simulink model "Simple_4Quad_payload_03"  (R2018b)
settings: Solver=VariableStepAuto  StartTime=0.0  StopTime=60  RelTol=1e-3
InitFcn:
  | Simple_4Quad_payload_03_const
values from neighbouring files (symbols this model uses):
  B = 1e0*eye(n)    [Simple_2Quad_payload_03_const.m]    (also in constant_CAMFC2_Quad_New_02_Payload_01.m = eye(n); test01.m = [eye(3) eye(3) eye(3) eye(3))
  BBT_inv = ((B'*B)^(-1))*B'    [Simple_2Quad_payload_03_const.m]    (also in Simple_4Quad_payload_04_const.m = ((BR'*BR)^(-1))*BR'; Simple_4Quad_payload_05_const.m = ((BR'*BR)^(-1))*BR'; Simple_4Quad_payload_06_const.m = ((BR'*BR)^(-1))*BR'; Simple_4Quad_payload_07_const.m = ((BR'*BR)^(-1))*BR')
  d1 = 0.25    [Colab_4Quad_model_01_const.m]    (also in Colab_4Quad_model_02_const.m = 0.5; Simple_4Quad_payload_01_const.m = 1; Simple_4Quad_payload_02_const.m = 1; Simple_4Quad_payload_03_const.m = 1)
  d2 = 0.25    [Colab_4Quad_model_01_const.m]    (also in Colab_4Quad_model_02_const.m = 0.5; Simple_4Quad_payload_01_const.m = 1; Simple_4Quad_payload_02_const.m = 1; Simple_4Quad_payload_03_const.m = 1)
  Des_rel_dist = 2    [Simple_4Quad_payload_01_const.m]    (also in Simple_4Quad_payload_02_const.m = 4; Simple_4Quad_payload_03_const.m = 4; Simple_4Quad_payload_04_const.m; Simple_4Quad_payload_05_const.m)
  gamma_0 = 1e-0*diag([1e-3;1e-0])    [Simple_2Quad_payload_03_const.m]    (also in Simple_4Quad_payload_04_const.m = 1e-0*diag([1e-6*ones(3,1);1e-0*ones(3,1)]); Simple_4Quad_payload_05_const.m = 1e-1*diag([1e-6*ones(3,1);1e-0*ones(3,1)]); Simple_4Quad_payload_06_const.m = 1e-0*diag([1e-6*ones(3,1);1e-0*ones(3,1)]); Simple_4Quad_payload_07_const.m = 1e-0*diag([1e-6*ones(3,1);1e-0*ones(3,1)]))
  gamma_1 = 1e+2*diag([1e-3;1e-0])    [Simple_2Quad_payload_03_const.m]    (also in Simple_4Quad_payload_04_const.m = 1e+2*diag([1e-6*ones(3,1);1e-0*ones(3,1)]); Simple_4Quad_payload_05_const.m = 1e+2*diag([1e-6*ones(3,1);1e-0*ones(3,1)]); Simple_4Quad_payload_06_const.m = 1e+3*diag([1e-6*ones(3,1);1e-0*ones(3,1)]); Simple_4Quad_payload_07_const.m = 1e+3*diag([1e-6*ones(3,1);1e-0*ones(3,1)]))
  ge = 9.81    [Simple_4Quad_payload_03_const.m]    (also in constant_CAMFC2_Quad_New_02_Payload_01.m)
  Ix = 0.166667    [Colab_4Quad_model_01_const.m]    (also in Colab_4Quad_model_02_const.m = 0.02; Simple_4Quad_payload_01_const.m = 1; Simple_4Quad_payload_02_const.m = 1; Simple_4Quad_payload_03_const.m = 1)
  Iy = 0.166667    [Colab_4Quad_model_01_const.m]    (also in Colab_4Quad_model_02_const.m = 0.02; Simple_4Quad_payload_01_const.m = 1; Simple_4Quad_payload_02_const.m = 1; Simple_4Quad_payload_03_const.m = 1)
  Iz = 0.166667    [Colab_4Quad_model_01_const.m]    (also in Colab_4Quad_model_02_const.m = 0.02; Simple_4Quad_payload_01_const.m = 1; Simple_4Quad_payload_02_const.m = 1; Simple_4Quad_payload_03_const.m = 1)
  Jq = diag([0.0291 0.0291 0.0552])    [Colab_4Quad_model_01_const.m]    (also in Colab_4Quad_model_02_const.m = diag([0.03 0.03 0.06]); Simple_4Quad_payload_03_const.m = 1.2416e-3 * diag([1 1 2]); Simple_4Quad_payload_04_const.m = 1 * diag([1 1 2]); Simple_4Quad_payload_05_const.m = 1 * diag([1 1 2]))
  k1 = 1    [Simple_2Quad_payload_03_const.m]    (also in Simple_4Quad_payload_04_const.m; Simple_4Quad_payload_05_const.m; Simple_4Quad_payload_06_const.m; Simple_4Quad_payload_07_const.m)
  k2 = 0.1    [Simple_2Quad_payload_03_const.m]    (also in Simple_4Quad_payload_04_const.m; Simple_4Quad_payload_05_const.m; Simple_4Quad_payload_06_const.m; Simple_4Quad_payload_07_const.m)
  Ka = 0.01    [Simple_4Quad_payload_03_const.m]    (also in constant_CAMFC2_Quad_New_02_Payload_01.m)
  Kd = 0.01    [Simple_4Quad_payload_03_const.m]    (also in constant_CAMFC2_Quad_New_02_Payload_01.m)
  Kf = 1.0e-5    (= 1e-05)    [Simple_4Quad_payload_03_const.m]    (also in constant_CAMFC2_Quad_New_02_Payload_01.m)
  ki1_N = 0    [Simple_4Quad_payload_02_const.m]    (also in Simple_4Quad_payload_03_const.m; Simple_4Quad_payload_04_const.m; Simple_4Quad_payload_05_const.m; Simple_4Quad_payload_06_const.m)
  ki1_S = 0    [Simple_4Quad_payload_02_const.m]    (also in Simple_4Quad_payload_03_const.m; Simple_4Quad_payload_04_const.m)
  ki2_N = 0    [Simple_4Quad_payload_02_const.m]    (also in Simple_4Quad_payload_03_const.m; Simple_4Quad_payload_04_const.m; Simple_4Quad_payload_05_const.m; Simple_4Quad_payload_06_const.m = 10)
  ki2_S = 0    [Simple_4Quad_payload_02_const.m]    (also in Simple_4Quad_payload_03_const.m; Simple_4Quad_payload_04_const.m)
  kp1_N = 10    [Simple_4Quad_payload_02_const.m]    (also in Simple_4Quad_payload_03_const.m; Simple_4Quad_payload_04_const.m; Simple_4Quad_payload_05_const.m = 1; Simple_4Quad_payload_06_const.m = 1)
  kp1_S = 10    [Simple_4Quad_payload_02_const.m]    (also in Simple_4Quad_payload_03_const.m; Simple_4Quad_payload_04_const.m)
  kp2_N = 100    [Simple_4Quad_payload_02_const.m]    (also in Simple_4Quad_payload_03_const.m; Simple_4Quad_payload_04_const.m; Simple_4Quad_payload_05_const.m = 1; Simple_4Quad_payload_06_const.m = 1)
  kp2_S = 100    [Simple_4Quad_payload_02_const.m]    (also in Simple_4Quad_payload_03_const.m; Simple_4Quad_payload_04_const.m)
  Kt = 0.0435 * Kf    (= 4.35e-07)    [Simple_4Quad_payload_03_const.m]    (also in constant_CAMFC2_Quad_New_02_Payload_01.m = 1e-07)
  l = 3.1819    [Colab_4Quad_model_01_const.m]    (also in Colab_4Quad_model_02_const.m = 3; Simple_2Quad_payload_04_const.m = 1; Simple_4Quad_payload_01_const.m = 1; Simple_4Quad_payload_02_const.m = 2)
  Lq = 0.45    [Simple_4Quad_payload_03_const.m]    (also in constant_CAMFC2_Quad_New_02_Payload_01.m = 0.2)
  m = 1.5    [Colab_4Quad_model_01_const.m]    (also in Colab_4Quad_model_02_const.m; Simple_2Quad_payload_04_const.m = 1; Simple_4Quad_payload_01_const.m = 1; Simple_4Quad_payload_02_const.m = 1)
  M = 1.0    (= 1)    [Colab_4Quad_model_01_const.m]    (also in Colab_4Quad_model_02_const.m; Simple_2Quad_payload_01_const.m; Simple_2Quad_payload_02_const.m; Simple_2Quad_payload_03_const.m)
  Md = 1*[1;1;1]    [Simple_2Quad_payload_04_const.m]    (also in Simple_4Quad_payload_01_const.m = 1*[1;1;1;1;1;1]; Simple_4Quad_payload_02_const.m = 1*[1;1;1;1;1;1]; Simple_4Quad_payload_03_const.m = 1*[1;1;1;1;1;1]; Simple_4Quad_payload_04_const.m = 1*[1;1;1;1;1;1])
  Mq = 2.95    [Simple_4Quad_payload_03_const.m]
  n = 2    [Simple_2Quad_payload_03_const.m]    (also in Simple_4Quad_payload_03_const.m = 6; Simple_4Quad_payload_04_const.m = 6; Simple_4Quad_payload_05_const.m = 6; Simple_4Quad_payload_06_const.m = 6)
  QR = 1e-0*eye(n)    [Simple_4Quad_payload_04_const.m]    (also in Simple_4Quad_payload_05_const.m = 1e-1*eye(n); Simple_4Quad_payload_06_const.m; Simple_4Quad_payload_07_const.m; Simple_4Quad_payload_08_const.m)
  R = 1e+0*eye(n)    [Simple_2Quad_payload_03_const.m]    (also in Simple_4Quad_payload_04_const.m = 1e+0*eye(m); Simple_4Quad_payload_05_const.m = 1e+0*eye(m); Simple_4Quad_payload_06_const.m; Simple_4Quad_payload_07_const.m)
  rho_0 = 1e-0    (= 1)    [Simple_2Quad_payload_03_const.m]    (also in Simple_4Quad_payload_04_const.m; Simple_4Quad_payload_05_const.m = 0.1; Simple_4Quad_payload_06_const.m; Simple_4Quad_payload_07_const.m)
  rho_1 = 1e-0    (= 1)    [Simple_2Quad_payload_03_const.m]    (also in Simple_4Quad_payload_04_const.m; Simple_4Quad_payload_05_const.m; Simple_4Quad_payload_06_const.m; Simple_4Quad_payload_07_const.m)
undefined symbols (not defined in the file or in its folder): mq
libraries: simulink x16
(part 3 of 3)

== matlab function Simple_4Quad_payload_03/Agent2/Quadrotor Plant #2/MATLAB Function ==
  data: XT2 input; XR2 input; Omega2_des input; t input; D_XT2 output; Kf parameter; Kt parameter; Kd parameter; Ka parameter; Mq parameter; Jq parameter; Lq parameter; ge parameter; D_XR2 output
function [D_XT2,D_XR2] = fcn(XT2,XR2,Omega2_des,t,Kf,Kt,Kd,Ka,Mq,Jq,Lq,ge)

phi_2 = XR2(1);
theta_2 = XR2(2);
psi_2 = XR2(3);

Rq_2 = [cos(psi_2)*cos(theta_2) -sin(psi_2)*cos(phi_2)+cos(psi_2)*sin(theta_2)*sin(phi_2) sin(psi_2)*sin(phi_2)+cos(psi_2)*sin(theta_2)*cos(phi_2);
    sin(psi_2)*cos(theta_2) cos(psi_2)*cos(phi_2)+sin(psi_2)*sin(theta_2)*sin(phi_2) -cos(psi_2)*sin(phi_2)+sin(psi_2)*sin(theta_2)*cos(phi_2);
    -sin(theta_2) cos(theta_2)*sin(phi_2) cos(theta_2)*cos(phi_2)]; 

R_omega_2 = [1 0 -sin(theta_2);
    0 cos(phi_2) cos(theta_2)*sin(phi_2);
    0 -sin(phi_2) cos(theta_2)*cos(phi_2)];

EXT_PRD_2 = External_Product3(XR2(4:6),(Jq*XR2(4:6)));

F1_2 = Kf * Omega2_des(1)^2;
F2_2 = Kf * Omega2_des(2)^2;
F3_2 = Kf * Omega2_des(3)^2;
F4_2 = Kf * Omega2_des(4)^2;
  
FT_2 = F1_2 + F2_2 + F3_2 + F4_2;
 
T1_2 = Kt * Omega2_des(1)^2;
T2_2 = Kt * Omega2_des(2)^2;
T3_2 = Kt * Omega2_des(3)^2;
T4_2 = Kt * Omega2_des(4)^2;
 
TT1_2 = Lq*(F3_2 - F1_2);
TT2_2 = Lq*(F4_2 - F2_2);
TT3_2 = (T1_2 - T2_2 + T3_2 - T4_2);

FTT_2 = Rq_2 * [0;0;FT_2];
FTx_2 = FTT_2(1);
FTy_2 = FTT_2(2);
FTz_2 = FTT_2(3);

DP_2 = XT2(4:6);
DPHI_2 = (R_omega_2)^(-1) * XR2(4:6); 
Dv_2 = (1/Mq)*([FTx_2;FTy_2;FTz_2] - Kd*XT2(4:6) - Mq*[0;0;ge]) + Rq_2*(0.0*sin(1*t))*[0;0;1]; 
Dw_2 = (Jq^(-1))*([TT1_2;TT2_2;TT3_2] - Ka*XR2(4:6) - EXT_PRD_2) + (0*sin(1*t)*[1;1;1]);

D_XT2 = [DP_2;Dv_2];
D_XR2 = [DPHI_2;Dw_2];

end

== matlab function Simple_4Quad_payload_03/Agent3/Attitude Controller #3/Rotational #3/CARE ==
  data: P input; a_hat input; B parameter; R parameter; DP output; QR parameter
function DP = fcn(P,a_hat,B,R,QR)

DP = a_hat*P + P*a_hat' - P*B*R*B'*P + 2*QR;

end

== matlab function Simple_4Quad_payload_03/Agent3/Attitude Controller #3/Rotational #3/Differentiator/Sliding differentiator ==
  data: u output; u1 input; e input; n parameter; k1 parameter
function u = fcn(u1,e,n,k1)

b=k1;

ABS = zeros(n,1);
for i=1:n
    if e(i)>0
        ABS(i) = e(i);
    else
        ABS(i) = -e(i);
    end
end
SGN = e ./ (ABS + 0.01);

u = u1 - b*(ABS.^0.5).*SGN;

end

== matlab function Simple_4Quad_payload_03/Agent3/Attitude Controller #3/Rotational #3/Differentiator/Sliding differentiator1 ==
  data: Du1 output; e input; n parameter; k2 parameter
function Du1 = fcn(e,n,k2)

a=k2;

ABS = zeros(n,1);
for i=1:n
    if e(i)>0
        ABS(i) = e(i);
    else
        ABS(i) = -e(i);
    end
end
SGN = e ./ (ABS + 0.01);

Du1 = - a*SGN;

end

== matlab function Simple_4Quad_payload_03/Agent3/Attitude Controller #3/Rotational #3/g-Estimator ==
  data: sigma input; g_hat input; P input; rho_1 parameter; gamma_1 parameter; Dg_hat output
function Dg_hat = fcn(sigma,g_hat,P,rho_1,gamma_1)

Dg_hat = - gamma_1 * P * sigma - rho_1 * gamma_1 * g_hat;

end

== matlab function Simple_4Quad_payload_03/Agent3/Attitude Controller #3/Rotational #3/g-Estimator1 ==
  data: sigma input; x input; P input; rho_0 parameter; gamma_0 parameter; Da_hat output; a_hat input
function Da_hat = fcn(sigma,x,P,rho_0,gamma_0,a_hat)

DVa_hat = - gamma_0 * P * diag(sigma) * (x - sigma) - rho_0 * gamma_0 * diag(a_hat);

Da_hat = diag(DVa_hat);

end

== matlab function Simple_4Quad_payload_03/Agent3/Attitude Controller #3/Rotational #3/main ==
  data: sigma input; zeta input; u output; Dy_d input; R parameter; P input; a_hat input; B parameter; g_hat input; x input; QR parameter; BBT_inv parameter; n parameter
function u = fcn(sigma,zeta,Dy_d,R,P,a_hat,B,g_hat,x,QR,BBT_inv,n)

u1 = (1/2) * R * B' * P * sigma;
u2 = BBT_inv * (Dy_d - a_hat*x + (eye(n) + 2*(((P)^(-1)*QR)) + a_hat)*sigma - g_hat - zeta) - (3/4) * R * B' * P * sigma;

u = u1 + u2;

end

== matlab function Simple_4Quad_payload_03/Agent3/Attitude Controller #3/Rotational #3/variable change ==
  data: X input; Xd input; x_mod output; u input; xd_mod output; e_mod output
function [x_mod,xd_mod,e_mod] = fcn(X,Xd,u)

x_mod = [X(4:6);X(10:12)];

xd_mod = [Xd;u(1:3)];

e_mod = xd_mod - x_mod;


end

== matlab function Simple_4Quad_payload_03/Agent3/Link angle computation #3 ==
  data: XT3 input; Alpha_act_3 output; Po input; Beta_act_3 output; PHIo input; L_meas_3 output
function [Alpha_act_3,Beta_act_3,L_meas_3] = fcn(XT3,Po,PHIo)

phi = PHIo(1);
theta = PHIo(2);
psi = PHIo(3);

Ro = [cos(psi)*cos(theta) cos(psi)*sin(theta)*sin(phi)-sin(psi)*cos(phi) cos(psi)*sin(theta)*cos(phi)+sin(psi)*sin(phi);
    sin(psi)*cos(theta) sin(psi)*sin(theta)*sin(phi)+cos(psi)*cos(phi) sin(psi)*sin(theta)*cos(phi)-cos(psi)*sin(phi);
    -sin(theta) cos(theta)*sin(phi) cos(theta)*cos(phi)];

P_diff_3 = Ro' * ( XT3(1:3) - Po );

L_meas_3 = sqrt( (P_diff_3(1)^2) + (P_diff_3(2)^2) + (P_diff_3(3)^2) );
Alpha_act_3 = asin( P_diff_3(3)/L_meas_3 );
Beta_act_3 = atan2( P_diff_3(2),P_diff_3(1) );
if Beta_act_3 < (-3*pi/4)
    Beta_act_3 = 2*pi + Beta_act_3;
end



end

== matlab function Simple_4Quad_payload_03/Agent3/Link dynamic Model #3 ==
  data: N3 input; S3 input; f3 input; alpha_3 input; beta_3 input; D_alpha_3 input; D_beta_3 input; mq parameter; ge parameter; DD_PHIo input; DD_Po input; D_PHIo input; l parameter; d2 parameter; PHIo input; U3_des output; Po input; P3_des output
function [U3_des,P3_des] = fcn(N3,S3,f3,alpha_3,beta_3,D_alpha_3,D_beta_3,mq,ge,DD_PHIo,DD_Po,D_PHIo, l, d2,PHIo,Po)

phi = PHIo(1);
theta = PHIo(2);
psi = PHIo(3);

Dist3_local = [0;+d2;0];
D3_angles = [0;D_alpha_3;D_beta_3];

Ro = [cos(psi)*cos(theta) cos(psi)*sin(theta)*sin(phi)-sin(psi)*cos(phi) cos(psi)*sin(theta)*cos(phi)+sin(psi)*sin(phi);
    sin(psi)*cos(theta) sin(psi)*sin(theta)*sin(phi)+cos(psi)*cos(phi) sin(psi)*sin(theta)*cos(phi)-cos(psi)*sin(phi);
    -sin(theta) cos(theta)*sin(phi) cos(theta)*cos(phi)];

R3 = [cos(alpha_3)*cos(beta_3) -sin(beta_3) -sin(alpha_3)*cos(beta_3);
    cos(alpha_3)*sin(beta_3) cos(beta_3) -sin(alpha_3)*sin(beta_3);
    sin(alpha_3) 0 cos(alpha_3)];

C1_3 = External_Product3(D_PHIo,Dist3_local);
C2_3 = External_Product3(D_PHIo,C1_3);
C3_3 = External_Product3(DD_PHIo,Dist3_local);
C4_3 = External_Product3(D3_angles,Dist3_local);
C5_3 = External_Product3(D3_angles,C4_3);

a3_part = (  R3' * ( Ro'*DD_Po + C2_3 + C3_3 ) ) + C5_3;
G3_local = R3' * Ro' * [0;0;-ge];

T3 = mq*a3_part(1) + f3 - mq*G3_local(1);
U3_des = Ro * R3 * [T3;S3;N3];

%DD_alpha3 = (1/mq/l) * (N3 - mq*a3_part(2) + mq*G3_local(2));
%DD_beta3 = (1/mq/l) * (S3 - mq*a3_part(3) + mq*G3_local(3));
P3_des = Po + Ro*Dist3_local + Ro*R3*[l;0;0];

end

== matlab function Simple_4Quad_payload_03/Agent3/Quadrotor Plant #3/MATLAB Function ==
  data: XT3 input; XR3 input; Omega3_des input; t input; D_XT3 output; Kf parameter; Kt parameter; Kd parameter; Ka parameter; Mq parameter; Jq parameter; Lq parameter; ge parameter; D_XR3 output
function [D_XT3,D_XR3] = fcn(XT3,XR3,Omega3_des,t,Kf,Kt,Kd,Ka,Mq,Jq,Lq,ge)

phi_3 = XR3(1);
theta_3 = XR3(2);
psi_3 = XR3(3);

Rq_3 = [cos(psi_3)*cos(theta_3) -sin(psi_3)*cos(phi_3)+cos(psi_3)*sin(theta_3)*sin(phi_3) sin(psi_3)*sin(phi_3)+cos(psi_3)*sin(theta_3)*cos(phi_3);
    sin(psi_3)*cos(theta_3) cos(psi_3)*cos(phi_3)+sin(psi_3)*sin(theta_3)*sin(phi_3) -cos(psi_3)*sin(phi_3)+sin(psi_3)*sin(theta_3)*cos(phi_3);
    -sin(theta_3) cos(theta_3)*sin(phi_3) cos(theta_3)*cos(phi_3)]; 

R_omega_3 = [1 0 -sin(theta_3);
    0 cos(phi_3) cos(theta_3)*sin(phi_3);
    0 -sin(phi_3) cos(theta_3)*cos(phi_3)];

EXT_PRD_3 = External_Product3(XR3(4:6),(Jq*XR3(4:6)));

F1_3 = Kf * Omega3_des(1)^2;
F2_3 = Kf * Omega3_des(2)^2;
F3_3 = Kf * Omega3_des(3)^2;
F4_3 = Kf * Omega3_des(4)^2;
  
FT_3 = F1_3 + F2_3 + F3_3 + F4_3;
 
T1_3 = Kt * Omega3_des(1)^2;
T2_3 = Kt * Omega3_des(2)^2;
T3_3 = Kt * Omega3_des(3)^2;
T4_3 = Kt * Omega3_des(4)^2;
 
TT1_3 = Lq*(F3_3 - F1_3);
TT2_3 = Lq*(F4_3 - F2_3);
TT3_3 = (T1_3 - T2_3 + T3_3 - T4_3);

FTT_3 = Rq_3 * [0;0;FT_3];
FTx_3 = FTT_3(1);
FTy_3 = FTT_3(2);
FTz_3 = FTT_3(3);

DP_3 = XT3(4:6);
DPHI_3 = (R_omega_3)^(-1) * XR3(4:6); 
Dv_3 = (1/Mq)*([FTx_3;FTy_3;FTz_3] - Kd*XT3(4:6) - Mq*[0;0;ge]) + Rq_3*(0.0*sin(1*t))*[0;0;1]; 
Dw_3 = (Jq^(-1))*([TT1_3;TT2_3;TT3_3] - Ka*XR3(4:6) - EXT_PRD_3) + (0*sin(1*t)*[1;1;1]);

D_XT3 = [DP_3;Dv_3];
D_XR3 = [DPHI_3;Dw_3];

end

== matlab function Simple_4Quad_payload_03/Agent4/Attitude Controller #4/Controller Interpreter #4 ==
  data: ut_4 input; uT_4 output; PHI_d_4 output
function [uT_4,PHI_d_4] = fcn(ut_4)

%%
fT_4 = sqrt((ut_4(1)^2)+(ut_4(2)^2)+(ut_4(3)^2));
psi_d_4 = 0;
phi_d_4 = asin( min(max(((sin(psi_d_4)*ut_4(1) - cos(psi_d_4)*ut_4(2)) / (fT_4+1e-3)),-1),1) );
theta_d_4 = atan( (cos(psi_d_4)*ut_4(1) + sin(psi_d_4)*ut_4(2)) / (ut_4(3)+1e-3) );
PHI_d_4 = [phi_d_4;theta_d_4;psi_d_4]; 
uT_4 = fT_4;

end

== matlab function Simple_4Quad_payload_03/Agent4/Attitude Controller #4/Controller to Motors #4 ==
  data: u_final_4 output; uT4 input; uR4 input; RM_1 parameter
function u_final_4 = fcn(uT4,uR4,RM_1)

y1_4 = uR4(4);
y2_4 = uR4(5);
y3_4 = uR4(6);

Y4 = [uT4;y1_4;y2_4;y3_4];

u_final_4 = RM_1*Y4;

for i=1:4
    u_final_4(i) = sqrt(abs(u_final_4(i)));
end

end

== matlab function Simple_4Quad_payload_03/Agent4/Attitude Controller #4/Rotational #4/CARE ==
  data: P input; a_hat input; B parameter; R parameter; DP output; QR parameter
function DP = fcn(P,a_hat,B,R,QR)

DP = a_hat*P + P*a_hat' - P*B*R*B'*P + 2*QR;

end

== matlab function Simple_4Quad_payload_03/Agent4/Attitude Controller #4/Rotational #4/Differentiator/Sliding differentiator ==
  data: u output; u1 input; e input; n parameter; k1 parameter
function u = fcn(u1,e,n,k1)

b=k1;

ABS = zeros(n,1);
for i=1:n
    if e(i)>0
        ABS(i) = e(i);
    else
        ABS(i) = -e(i);
    end
end
SGN = e ./ (ABS + 0.01);

u = u1 - b*(ABS.^0.5).*SGN;

end

== matlab function Simple_4Quad_payload_03/Agent4/Attitude Controller #4/Rotational #4/Differentiator/Sliding differentiator1 ==
  data: Du1 output; e input; n parameter; k2 parameter
function Du1 = fcn(e,n,k2)

a=k2;

ABS = zeros(n,1);
for i=1:n
    if e(i)>0
        ABS(i) = e(i);
    else
        ABS(i) = -e(i);
    end
end
SGN = e ./ (ABS + 0.01);

Du1 = - a*SGN;

end

== matlab function Simple_4Quad_payload_03/Agent4/Attitude Controller #4/Rotational #4/g-Estimator ==
  data: sigma input; g_hat input; P input; rho_1 parameter; gamma_1 parameter; Dg_hat output
function Dg_hat = fcn(sigma,g_hat,P,rho_1,gamma_1)

Dg_hat = - gamma_1 * P * sigma - rho_1 * gamma_1 * g_hat;

end

== matlab function Simple_4Quad_payload_03/Agent4/Attitude Controller #4/Rotational #4/g-Estimator1 ==
  data: sigma input; x input; P input; rho_0 parameter; gamma_0 parameter; Da_hat output; a_hat input
function Da_hat = fcn(sigma,x,P,rho_0,gamma_0,a_hat)

DVa_hat = - gamma_0 * P * diag(sigma) * (x - sigma) - rho_0 * gamma_0 * diag(a_hat);

Da_hat = diag(DVa_hat);

end

== matlab function Simple_4Quad_payload_03/Agent4/Attitude Controller #4/Rotational #4/main ==
  data: sigma input; zeta input; u output; Dy_d input; R parameter; P input; a_hat input; B parameter; g_hat input; x input; QR parameter; BBT_inv parameter; n parameter
function u = fcn(sigma,zeta,Dy_d,R,P,a_hat,B,g_hat,x,QR,BBT_inv,n)

u1 = (1/2) * R * B' * P * sigma;
u2 = BBT_inv * (Dy_d - a_hat*x + (eye(n) + 2*(((P)^(-1)*QR)) + a_hat)*sigma - g_hat - zeta) - (3/4) * R * B' * P * sigma;

u = u1 + u2;

end

== matlab function Simple_4Quad_payload_03/Agent4/Attitude Controller #4/Rotational #4/variable change ==
  data: X input; Xd input; x_mod output; u input; xd_mod output; e_mod output
function [x_mod,xd_mod,e_mod] = fcn(X,Xd,u)

x_mod = [X(4:6);X(10:12)];

xd_mod = [Xd;u(1:3)];

e_mod = xd_mod - x_mod;


end

== matlab function Simple_4Quad_payload_03/Agent4/Link angle computation #4 ==
  data: XT4 input; Alpha_act_4 output; Po input; Beta_act_4 output; PHIo input; L_meas_4 output
function [Alpha_act_4,Beta_act_4,L_meas_4] = fcn(XT4,Po,PHIo)

phi = PHIo(1);
theta = PHIo(2);
psi = PHIo(3);

Ro = [cos(psi)*cos(theta) cos(psi)*sin(theta)*sin(phi)-sin(psi)*cos(phi) cos(psi)*sin(theta)*cos(phi)+sin(psi)*sin(phi);
    sin(psi)*cos(theta) sin(psi)*sin(theta)*sin(phi)+cos(psi)*cos(phi) sin(psi)*sin(theta)*cos(phi)-cos(psi)*sin(phi);
    -sin(theta) cos(theta)*sin(phi) cos(theta)*cos(phi)];

P_diff_4 = Ro' * ( XT4(1:3) - Po );

L_meas_4 = sqrt( (P_diff_4(1)^2) + (P_diff_4(2)^2) + (P_diff_4(3)^2) );
Alpha_act_4 = asin( P_diff_4(3)/L_meas_4 );
Beta_act_4 = atan2( P_diff_4(2),P_diff_4(1) );
if Beta_act_4 < (-3*pi/4)
    Beta_act_4 = 2*pi + Beta_act_43;
end



end

== matlab function Simple_4Quad_payload_03/Agent4/Link dynamic Model #4 ==
  data: N4 input; S4 input; f4 input; alpha_4 input; beta_4 input; D_alpha_4 input; D_beta_4 input; mq parameter; ge parameter; DD_PHIo input; DD_Po input; D_PHIo input; l parameter; d2 parameter; PHIo input; U4_des output; Po input; P4_des output
function [U4_des,P4_des] = fcn(N4,S4,f4,alpha_4,beta_4,D_alpha_4,D_beta_4,mq,ge,DD_PHIo,DD_Po,D_PHIo, l, d2,PHIo,Po)

phi = PHIo(1);
theta = PHIo(2);
psi = PHIo(3);

Dist4_local = [0;-d2;0];
D4_angles = [0;D_alpha_4;D_beta_4];

Ro = [cos(psi)*cos(theta) cos(psi)*sin(theta)*sin(phi)-sin(psi)*cos(phi) cos(psi)*sin(theta)*cos(phi)+sin(psi)*sin(phi);
    sin(psi)*cos(theta) sin(psi)*sin(theta)*sin(phi)+cos(psi)*cos(phi) sin(psi)*sin(theta)*cos(phi)-cos(psi)*sin(phi);
    -sin(theta) cos(theta)*sin(phi) cos(theta)*cos(phi)];

R4 = [cos(alpha_4)*cos(beta_4) -sin(beta_4) -sin(alpha_4)*cos(beta_4);
    cos(alpha_4)*sin(beta_4) cos(beta_4) -sin(alpha_4)*sin(beta_4);
    sin(alpha_4) 0 cos(alpha_4)];

C1_4 = External_Product3(D_PHIo,Dist4_local);
C2_4 = External_Product3(D_PHIo,C1_4);
C3_4 = External_Product3(DD_PHIo,Dist4_local);
C4_4 = External_Product3(D4_angles,Dist4_local);
C5_4 = External_Product3(D4_angles,C4_4);

a4_part = (  R4' * ( Ro'*DD_Po + C2_4 + C3_4 ) ) + C5_4;
G4_local = R4' * Ro' * [0;0;-ge];

T4 = mq*a4_part(1) + f4 - mq*G4_local(1);
U4_des = Ro * R4 * [T4;S4;N4];

%DD_alpha4 = (1/mq/l) * (N4 - mq*a4_part(2) + mq*G4_local(2));
%DD_beta4 = (1/mq/l) * (S4 - mq*a4_part(3) + mq*G4_local(3));
P4_des = Po + Ro*Dist4_local + Ro*R4*[l;0;0];

end

== matlab function Simple_4Quad_payload_03/Agent4/Quadrotor Plant #4/MATLAB Function ==
  data: XT4 input; XR4 input; Omega4_des input; t input; D_XT4 output; Kf parameter; Kt parameter; Kd parameter; Ka parameter; Mq parameter; Jq parameter; Lq parameter; ge parameter; D_XR4 output
function [D_XT4,D_XR4] = fcn(XT4,XR4,Omega4_des,t,Kf,Kt,Kd,Ka,Mq,Jq,Lq,ge)

phi_4 = XR4(1);
theta_4 = XR4(2);
psi_4 = XR4(3);

Rq_4 = [cos(psi_4)*cos(theta_4) -sin(psi_4)*cos(phi_4)+cos(psi_4)*sin(theta_4)*sin(phi_4) sin(psi_4)*sin(phi_4)+cos(psi_4)*sin(theta_4)*cos(phi_4);
    sin(psi_4)*cos(theta_4) cos(psi_4)*cos(phi_4)+sin(psi_4)*sin(theta_4)*sin(phi_4) -cos(psi_4)*sin(phi_4)+sin(psi_4)*sin(theta_4)*cos(phi_4);
    -sin(theta_4) cos(theta_4)*sin(phi_4) cos(theta_4)*cos(phi_4)]; 

R_omega_4 = [1 0 -sin(theta_4);
    0 cos(phi_4) cos(theta_3)*sin(phi_4);
    0 -sin(phi_4) cos(theta_3)*cos(phi_4)];

EXT_PRD_4 = External_Product3(XR4(4:6),(Jq*XR4(4:6)));

F1_4 = Kf * Omega4_des(1)^2;
F2_4 = Kf * Omega4_des(2)^2;
F3_4 = Kf * Omega4_des(3)^2;
F4_4 = Kf * Omega4_des(4)^2;
  
FT_4 = F1_4 + F2_4 + F3_4 + F4_4;
 
T1_4 = Kt * Omega4_des(1)^2;
T2_4 = Kt * Omega4_des(2)^2;
T3_4 = Kt * Omega4_des(3)^2;
T4_4 = Kt * Omega4_des(4)^2;
 
TT1_4 = Lq*(F3_4 - F1_4);
TT2_4 = Lq*(F4_4 - F2_4);
TT3_4 = (T1_4 - T2_4 + T3_4 - T4_4);

FTT_4 = Rq_4 * [0;0;FT_4];
FTx_4 = FTT_4(1);
FTy_4 = FTT_4(2);
FTz_4 = FTT_4(3);

DP_4 = XT4(4:6);
DPHI_4 = (R_omega_4)^(-1) * XR4(4:6); 
Dv_4 = (1/Mq)*([FTx_4;FTy_4;FTz_4] - Kd*XT4(4:6) - Mq*[0;0;ge]) + Rq_4*(0.0*sin(1*t))*[0;0;1]; 
Dw_4 = (Jq^(-1))*([TT1_4;TT2_4;TT3_4] - Ka*XR4(4:6) - EXT_PRD_4) + (0*sin(1*t)*[1;1;1]);

D_XT4 = [DP_4;Dv_4];
D_XR4 = [DPHI_4;Dw_4];

end

== matlab function Simple_4Quad_payload_03/Agent1 /Attitude Controller #1/Rotational #1/CARE ==
  data: P input; a_hat input; B parameter; R parameter; DP output; QR parameter
function DP = fcn(P,a_hat,B,R,QR)

DP = a_hat*P + P*a_hat' - P*B*R*B'*P + 2*QR;

end

== matlab function Simple_4Quad_payload_03/Agent1 /Attitude Controller #1/Rotational #1/Differentiator/Sliding differentiator ==
  data: u output; u1 input; e input; n parameter; k1 parameter
function u = fcn(u1,e,n,k1)

b=k1;

ABS = zeros(n,1);
for i=1:n
    if e(i)>0
        ABS(i) = e(i);
    else
        ABS(i) = -e(i);
    end
end
SGN = e ./ (ABS + 0.01);

u = u1 - b*(ABS.^0.5).*SGN;

end

== matlab function Simple_4Quad_payload_03/Agent1 /Attitude Controller #1/Controller Interpreter #1 ==
  data: ut_1 input; uT_1 output; PHI_d_1 output
function [uT_1,PHI_d_1] = fcn(ut_1)

%%
fT_1 = sqrt((ut_1(1)^2)+(ut_1(2)^2)+(ut_1(3)^2));
psi_d_1 = 0;
phi_d_1 = asin( min(max(((sin(psi_d_1)*ut_1(1) - cos(psi_d_1)*ut_1(2)) / (fT_1+1e-3)),-1),1) );
theta_d_1 = atan( (cos(psi_d_1)*ut_1(1) + sin(psi_d_1)*ut_1(2)) / (ut_1(3)+1e-3) );
PHI_d_1 = [phi_d_1;theta_d_1;psi_d_1]; 
uT_1 = fT_1;

end

== matlab function Simple_4Quad_payload_03/Agent1 /Attitude Controller #1/Rotational #1/Differentiator/Sliding differentiator1 ==
  data: Du1 output; e input; n parameter; k2 parameter
function Du1 = fcn(e,n,k2)

a=k2;

ABS = zeros(n,1);
for i=1:n
    if e(i)>0
        ABS(i) = e(i);
    else
        ABS(i) = -e(i);
    end
end
SGN = e ./ (ABS + 0.01);

Du1 = - a*SGN;

end

== matlab function Simple_4Quad_payload_03/Agent1 /Attitude Controller #1/Rotational #1/g-Estimator ==
  data: sigma input; g_hat input; P input; rho_1 parameter; gamma_1 parameter; Dg_hat output
function Dg_hat = fcn(sigma,g_hat,P,rho_1,gamma_1)

Dg_hat = - gamma_1 * P * sigma - rho_1 * gamma_1 * g_hat;

end

== matlab function Simple_4Quad_payload_03/Agent1 /Attitude Controller #1/Rotational #1/g-Estimator1 ==
  data: sigma input; x input; P input; rho_0 parameter; gamma_0 parameter; Da_hat output; a_hat input
function Da_hat = fcn(sigma,x,P,rho_0,gamma_0,a_hat)

DVa_hat = - gamma_0 * P * diag(sigma) * (x - sigma) - rho_0 * gamma_0 * diag(a_hat);

Da_hat = diag(DVa_hat);

end

== matlab function Simple_4Quad_payload_03/Agent1 /Attitude Controller #1/Rotational #1/main ==
  data: sigma input; zeta input; u output; Dy_d input; R parameter; P input; a_hat input; B parameter; g_hat input; x input; QR parameter; BBT_inv parameter; n parameter
function u = fcn(sigma,zeta,Dy_d,R,P,a_hat,B,g_hat,x,QR,BBT_inv,n)

u1 = (1/2) * R * B' * P * sigma;
u2 = BBT_inv * (Dy_d - a_hat*x + (eye(n) + 2*(((P)^(-1)*QR)) + a_hat)*sigma - g_hat - zeta) - (3/4) * R * B' * P * sigma;

u = u1 + u2;

end

== matlab function Simple_4Quad_payload_03/Agent1 /Attitude Controller #1/Rotational #1/variable change ==
  data: X input; Xd input; x_mod output; u input; xd_mod output; e_mod output
function [x_mod,xd_mod,e_mod] = fcn(X,Xd,u)

x_mod = [X(4:6);X(10:12)];

xd_mod = [Xd;u(1:3)];

e_mod = xd_mod - x_mod;


end
